simulink model "TS05_prevodova_mer"  (R2022b)
settings: Solver=ode45  StartTime=0.0  StopTime=60*4*11  RelTol=1e-3  EnableMultiTasking=on
undefined symbols (not defined in the file or in its folder): Advantech, PCI
libraries: sldrtlib x4
settings Model: Creator=Admin  LastModifiedBy=admin
settings SolverCC: AlgebraicLoopSolver=TrustRegion
settings DataIOCC: LimitDataPoints=on  SaveFormat=Array  ReturnWorkspaceOutputs=off
settings OptimizationCC: LifeSpan=inf
settings DebuggingCC: UnconnectedInputMsg=warning  UnconnectedOutputMsg=warning  UnconnectedLineMsg=warning  SFUnexpectedBacktrackingDiag=warning  SFNoUnconditionalDefaultTransitionDiag=warning  SFExecutionAtInitializationDiag=none  SFMachineParentedDataDiag=warning  ArithmeticOperatorsInVariantConditions=warning
settings HardwareCC: ProdBitPerPointer=32  ProdBitPerSizeT=32  ProdBitPerPtrDiffT=32  ProdLargestAtomicFloat=None  ProdIntDivRoundTo=Undefined  ProdEndianess=Unspecified  ProdWordSize=32  ProdHWDeviceType=32-bit Generic
settings ModelReferenceCC: PropagateSignalLabelsOutOfModel=off
settings SFSimCC: SimUseLocalCustomCode=off  CustomCodeUndefinedFunction=UseInterfaceOnly
settings RTWCC: RTWUseLocalCustomCode=off
settings CodeAppCC: StateflowObjectComments=on
settings GRTTargetCC: TargetLangStandard=C89/C90 (ANSI)
settings ConfigComp: CovMetricSettings=dw  CovSaveCumulativeToWorkspaceVar=on  CovSaveSingleToWorkspaceVar=on  CovExternalEMLEnable=off

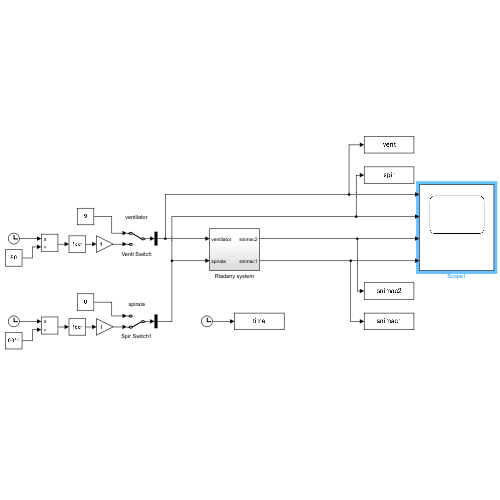
[thumbnail: Simulink's stored preview of the top-level diagram]
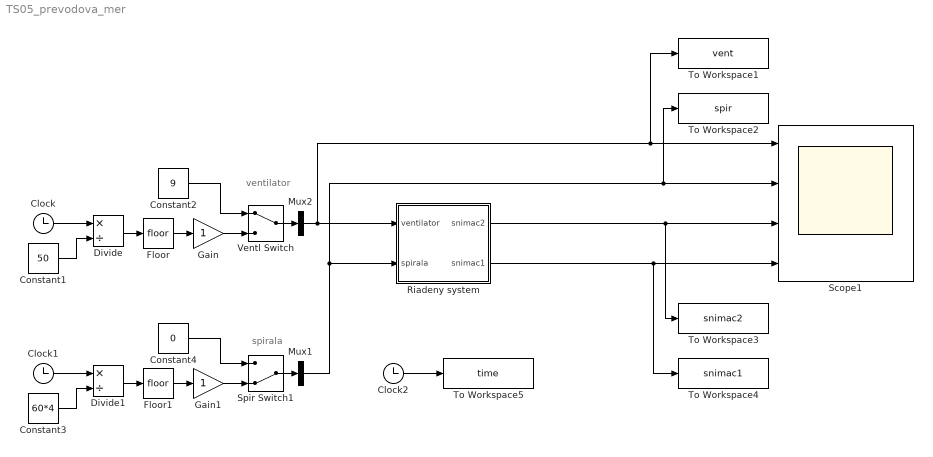
== system TS05_prevodova_mer ==
  note: spirala
  note: ventilator
  Clock : Clock
  Clock1 : Clock
  Clock2 : Clock
  Constant1 : Constant  Value=50
  Constant2 : Constant  Value=9
  Constant3 : Constant  Value=60*4
  Constant4 : Constant  Value=0
  Divide : Product  Inputs=*/
  Divide1 : Product  Inputs=*/
  Floor : Rounding
  Floor1 : Rounding
  Gain : Gain
  Gain1 : Gain
  Mux1 : Mux  Inputs=1
  Mux2 : Mux  Inputs=1
  Riadeny system : Subsystem
  Scope1 : Scope  NumInputPorts=4
  Spir Switch1 : ManualSwitch  CurrentSetting=0
  To Workspace1 : ToWorkspace  VariableName=vent  SampleTime=0.1
      settings: Save2DSignal=2-D array (concatenate along first dimension)
  To Workspace2 : ToWorkspace  VariableName=spir  SampleTime=0.1
      settings: Save2DSignal=2-D array (concatenate along first dimension)
  To Workspace3 : ToWorkspace  VariableName=snimac2  SampleTime=0.1
      settings: Save2DSignal=2-D array (concatenate along first dimension)
  To Workspace4 : ToWorkspace  VariableName=snimac1  SampleTime=0.1
      settings: Save2DSignal=2-D array (concatenate along first dimension)
  To Workspace5 : ToWorkspace  VariableName=time  SampleTime=0.1
      settings: Save2DSignal=2-D array (concatenate along first dimension)
  Ventl Switch : ManualSwitch
  wires:
  Mux2/1 -> Riadeny system/1(ventilator), To Workspace1/1, Scope1/1
  Riadeny system/1(snimac2) -> To Workspace3/1, Scope1/3
  Riadeny system/2(snimac1) -> To Workspace4/1, Scope1/4
  Mux1/1 -> Riadeny system/2(spirala), To Workspace2/1, Scope1/2
  Floor/1 -> Gain/1
  Clock/1 -> Divide/1
  Constant1/1 -> Divide/2
  Divide/1 -> Floor/1
  Ventl Switch/1 -> Mux2/1
  Constant2/1 -> Ventl Switch/1
  Gain/1 -> Ventl Switch/2
  Gain1/1 -> Spir Switch1/2
  Constant4/1 -> Spir Switch1/1
  Floor1/1 -> Gain1/1
  Constant3/1 -> Divide1/2
  Divide1/1 -> Floor1/1
  Clock1/1 -> Divide1/1
  Spir Switch1/1 -> Mux1/1
  Clock2/1 -> To Workspace5/1

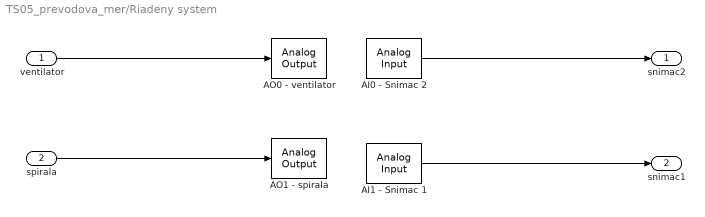
== system TS05_prevodova_mer/Riadeny system ==
  ventilator : Inport
  spirala : Inport  Port=2
  AI0 - Snimac 2 : sldrtlib/Analog Input  SampleTime=0.1  MaxMissedTicks=10  ShowMissedTicks=off  YieldWhenWaiting=off  DrvName=Advantech/PCI-1711  DrvAddress=4294967295  DrvOptions=zeros(1,0)  Channels=1  RangeMode=1  VoltRange=1  DataType=1
      settings: AttributesFormatString=Advantech\nPCI-1711 [auto]
  AI1 - Snimac 1 : sldrtlib/Analog Input  SampleTime=0.1  MaxMissedTicks=10  ShowMissedTicks=off  YieldWhenWaiting=off  DrvName=Advantech/PCI-1711  DrvAddress=4294967295  DrvOptions=zeros(1,0)  Channels=2  RangeMode=1  VoltRange=1  DataType=1
      settings: AttributesFormatString=Advantech\nPCI-1711 [auto]
  AO0 - ventilator : sldrtlib/Analog Output  SampleTime=0.1  MaxMissedTicks=10  ShowMissedTicks=off  YieldWhenWaiting=off  DrvName=Advantech/PCI-1711  DrvAddress=4294967295  DrvOptions=zeros(1,0)  Channels=1  RangeMode=1  VoltRange=2  InitialValue=[]  FinalValue=[]
      settings: AttributesFormatString=Advantech\nPCI-1711 [auto]
  AO1 - spirala : sldrtlib/Analog Output  SampleTime=0.1  MaxMissedTicks=10  ShowMissedTicks=off  YieldWhenWaiting=off  DrvName=Advantech/PCI-1711  DrvAddress=4294967295  DrvOptions=zeros(1,0)  Channels=2  RangeMode=1  VoltRange=2  InitialValue=[]  FinalValue=[]
      settings: AttributesFormatString=Advantech\nPCI-1711 [auto]
  snimac2 : Outport
  snimac1 : Outport  Port=2
  wires:
  ventilator/1 -> AO0 - ventilator/1
  spirala/1 -> AO1 - spirala/1
  AI1 - Snimac 1/1 -> snimac1/1
  AI0 - Snimac 2/1 -> snimac2/1
